simulink model "pi_control_with_disturbance"  (R2023b)
settings: Solver=VariableStepAuto  StartTime=0.0  StopTime=20  RelTol=1e-3
libraries: simulink x2
settings Model: Creator=kijun  LastModifiedBy=kijun

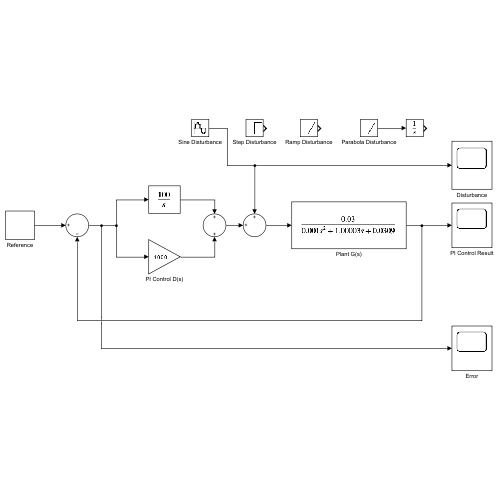
[thumbnail: Simulink's stored preview of the top-level diagram]
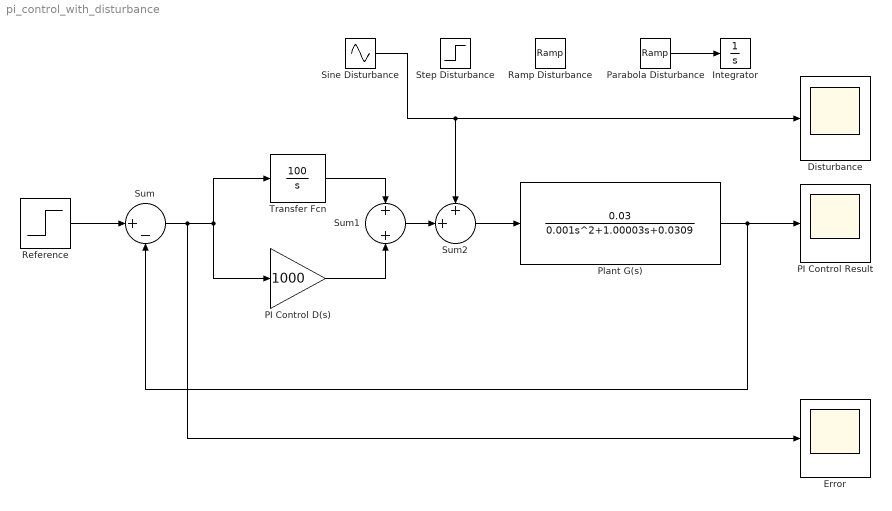
== system pi_control_with_disturbance ==
  Disturbance : Scope
  Error : Scope
  Integrator : Integrator
  PI Control D(s) : Gain  Gain=1000
  PI Control Result : Scope
  Parabola Disturbance : simulink/Sources/Ramp  slope=10  start=0  InitialOutput=0
  Plant G(s) : TransferFcn  Numerator=[0.03]  Denominator=[0.001 1.00003 0.0309]
  Ramp Disturbance : simulink/Sources/Ramp  slope=1  start=0  InitialOutput=0
  Reference : Step  Time=0  SampleTime=0
  Sine Disturbance : Sin  Bias=5  Frequency=5  SampleTime=0.001
  Step Disturbance : Step  Time=0  SampleTime=0
  Sum : Sum  Inputs=|+-
  Sum1 : Sum  Inputs=+|+
  Sum2 : Sum  Inputs=++|
  Transfer Fcn : TransferFcn  Numerator=100  Denominator=[1 0]
  wires:
  Sum1/1 -> Sum2/2
  Sum/1 -> Error/1, PI Control D(s)/1, Transfer Fcn/1
  Transfer Fcn/1 -> Sum1/1
  Plant G(s)/1 -> PI Control Result/1, Sum/2
  PI Control D(s)/1 -> Sum1/2
  Sum2/1 -> Plant G(s)/1
  Parabola Disturbance/1 -> Integrator/1
  Sine Disturbance/1 -> Disturbance/1, Sum2/1
  Reference/1 -> Sum/1
